simulink model "pendulo"  (R2025b)
settings: Solver=VariableStepAuto  StartTime=0.0  StopTime=10  RelTol=1e-3
settings Model: Creator=Gibra  LastModifiedBy=Gibra

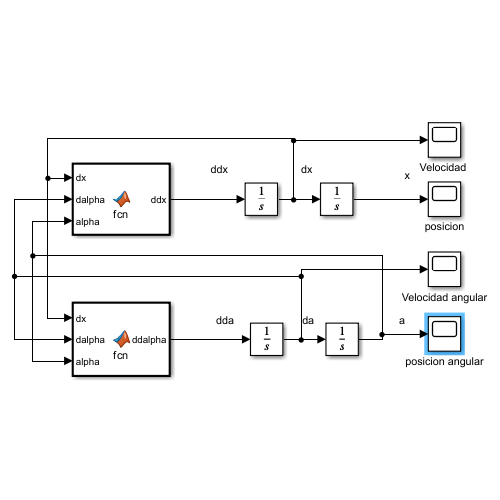
[thumbnail: Simulink's stored preview of the top-level diagram]
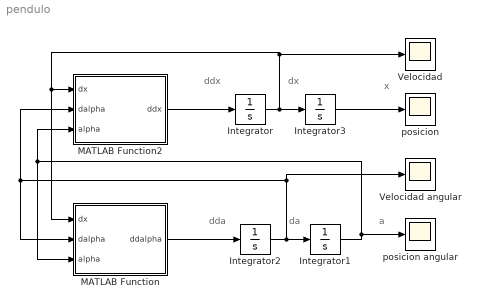
== system pendulo ==
  note: ddx
  note: dx
  note: x
  note: dda
  note: da
  note: a
  Integrator : Integrator
  Integrator1 : Integrator
  Integrator2 : Integrator  InitialCondition=1
  Integrator3 : Integrator
  MATLAB Function : MATLAB Function  TreatAsAtomicUnit=on
  MATLAB Function2 : MATLAB Function  TreatAsAtomicUnit=on
  "Velocidad " : Scope
      settings: ActiveDisplayYMinimum=-0.67063847356867412  ActiveDisplayYMaximum=0.59931739569261366  DataLoggingVariableName=ScopeData3
  Velocidad angular : Scope
      settings: ActiveDisplayYMinimum=-1  ActiveDisplayYMaximum=1
  posicion : Scope
      settings: ActiveDisplayYMinimum=-0.11641528655880171  ActiveDisplayYMaximum=0.2477918033441362
  posicion angular : Scope
      settings: ActiveDisplayYMinimum=-0.656106498864083  ActiveDisplayYMaximum=5.9049584897767478  DataLoggingVariableName=ScopeData2
  wires:
  Integrator2/1 -> MATLAB Function/2(dalpha), MATLAB Function2/2(dalpha), Velocidad angular/1, Integrator1/1
  Integrator/1 -> "Velocidad "/1, MATLAB Function/1(dx), MATLAB Function2/1(dx), Integrator3/1
  MATLAB Function2/1(ddx) -> Integrator/1
  Integrator1/1 -> MATLAB Function/3(alpha), MATLAB Function2/3(alpha), posicion angular/1
  MATLAB Function/1(ddalpha) -> Integrator2/1
  Integrator3/1 -> posicion/1

== matlab function pendulo/MATLAB Function2 ==
  data: dx input; ddx output; dalpha input; alpha input
function ddx = fcn(dx, dalpha, alpha)
    Ip = 0.0079;
    Mc = 0.7031;
    lp = 0.3302;
    Mp = 0.23;
    Fc = 0;
    Beq = 4.3;
    g = 9.81;
    Bp = 0.0024;
    ddx = ( (Ip + Mp*lp^2)*Fc + Mp^2*lp^2*g*cos(alpha)*sin(alpha) - (Ip + Mp*lp^2)*Beq*dx - (Ip*Mp*lp + Mp^2*lp^3)*dalpha^2*sin(alpha) - Mp*lp*dalpha*cos(alpha)*Bp) / ( (Mc + Mp)*Ip + Mc*Mp*lp^2 + Mp^2*lp^2*sin(alpha)^2 );

== matlab function pendulo/MATLAB Function ==
  data: dx input; ddalpha output; dalpha input; alpha input
function ddalpha = fcn(dx, dalpha, alpha)
   Ip = 0.0079;
    Mc = 0.7031;
    lp = 0.3302;
    Mp = 0.23;
    Fc = 0;
    Beq = 4.3;
    g = 9.81;
    Bp = 0.0024;
    ddalpha = ((Mc + Mp) * Mp * g * lp * sin(alpha) - (Mc + Mp) * Bp * dalpha + Fc * Mp * lp * cos(alpha) - Mp^2 *lp^2 * dalpha^2 * sin(alpha) * cos(alpha) - Beq * Mp * lp * dx * cos(alpha)) / ((Mc + Mp) * Ip + Mc * Mp * lp^2 + Mp^2 * lp^2 * sin(alpha)^2);
